simulink model "simulink_model_closed_loop"  (R2022b)
settings: Solver=ode45  StartTime=0.0  StopTime=1  RelTol=1e-3
values from neighbouring files (symbols this model uses):
  N = 20    [run_simulink.m]
  nu = 1    [run_simulink.m]
  ny = nx+nu    (= 5)    [run_simulink.m]
  ny_e = nx    (= 4)    [run_simulink.m]
  U_max = 40    [run_simulink.m]
  x0 = [0.0, 0.15*pi, 0.0, 0.0]    [run_simulink.m]
settings Model: Creator=oj  LastModifiedBy=amon
settings SolverCC: AlgebraicLoopSolver=TrustRegion
settings DataIOCC: SaveFormat=StructureWithTime
settings OptimizationCC: LifeSpan=inf
settings DebuggingCC: UnconnectedInputMsg=warning  UnconnectedOutputMsg=warning  UnconnectedLineMsg=warning  SFExecutionAtInitializationDiag=none  SFMachineParentedDataDiag=warning  ArithmeticOperatorsInVariantConditions=warning
settings HardwareCC: ProdBitPerSizeT=32  ProdBitPerPtrDiffT=32  ProdWordSize=32  ProdHWDeviceType=Specified
settings SFSimCC: CustomCodeUndefinedFunction=UseInterfaceOnly
settings CodeAppCC: StateflowObjectComments=on

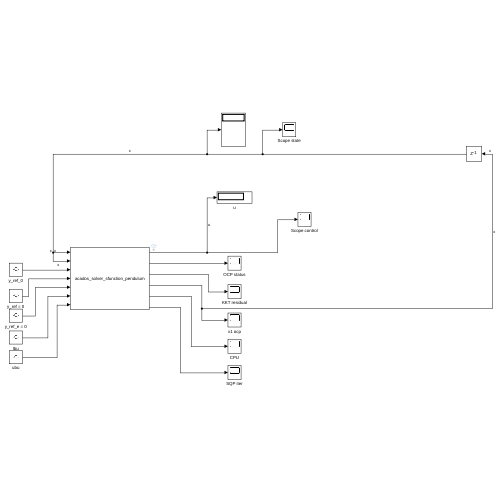
[thumbnail: Simulink's stored preview of the top-level diagram]
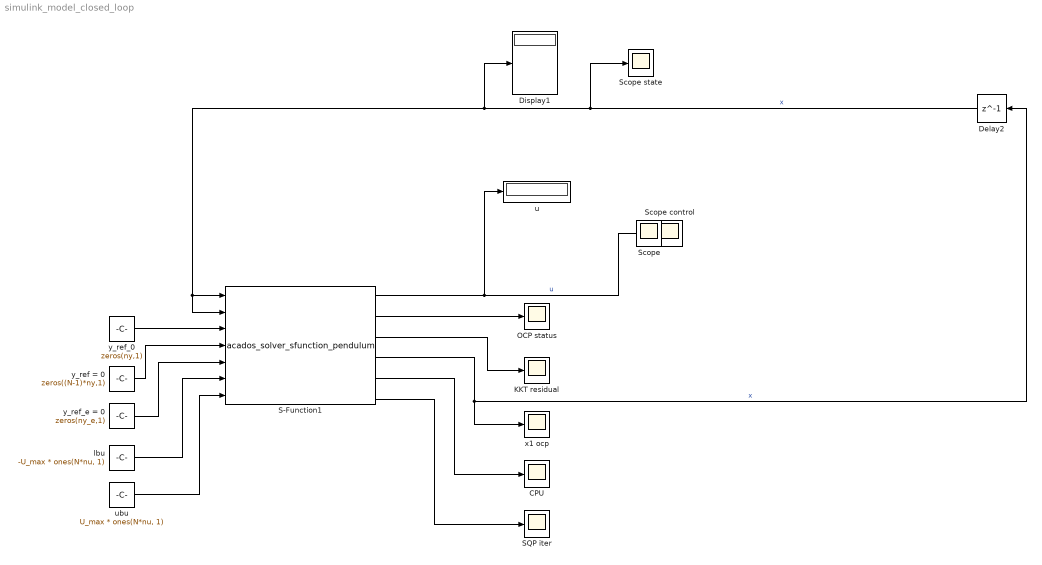
== system simulink_model_closed_loop ==
  CPU : Scope
      settings: Description=status
  Delay2 : Delay  DelayLength=1  InitialCondition=x0
  Display1 : Display
  KKT residual : Scope
      settings: Description=status
  OCP status : Scope
      settings: Description=status
  S-Function1 : S-Function  FunctionName=acados_solver_sfunction_pendulum  SFunctionDeploymentMode=off  EnableBusSupport=off
  SQP iter : Scope
      settings: Description=status
  Scope control : Scope
  Scope state : Scope
  lbu : Constant  Value=-U_max * ones(N*nu, 1)
  u : Display
  ubu : Constant  Value=U_max * ones(N*nu, 1)
  x1 ocp : Scope
      settings: Description=status
  y_ref = 0 : Constant  Value=zeros((N-1)*ny,1)
  y_ref_0 : Constant  Value=zeros(ny,1)
  y_ref_e = 0 : Constant  Value=zeros(ny_e,1)
  Scope : Scope
  wires:
  S-Function1/4 -> x1 ocp/1, Delay2/1  "x"
  S-Function1/2 -> OCP status/1
  S-Function1/3 -> KKT residual/1
  S-Function1/5 -> CPU/1
  lbu/1 -> S-Function1/6
  S-Function1/1 -> u/1, Scope control/1  "u"
  Delay2/1 -> S-Function1/2, S-Function1/1, Display1/1, Scope state/1  "x"
  S-Function1/6 -> SQP iter/1
  ubu/1 -> S-Function1/7
  y_ref_e = 0/1 -> S-Function1/5
  y_ref = 0/1 -> S-Function1/4
  y_ref_0/1 -> S-Function1/3
